simulink library "MOT_lib"  (R2016b)
settings: Solver=ode45  StartTime=0.0  StopTime=10.0  RelTol=1e-3  EnableMultiTasking=on
values from neighbouring files (symbols this model uses):
  MOT = MOTmod    [setup_mot.m]    (also in setup_motor.m)
undefined symbols (not defined in the file or in its folder): DiscIntNeverNeededParam
libraries: aerolibutil x1, aerolibtransform2 x1
settings Model: Creator=Andrew  LastModifiedBy=Andrew
settings DataIOCC: LimitDataPoints=on  SaveFormat=Array
settings OptimizationCC: LifeSpan=inf
settings DebuggingCC: SFUnexpectedBacktrackingDiag=warning  SFNoUnconditionalDefaultTransitionDiag=warning  SFExecutionAtInitializationDiag=none
settings HardwareCC: ProdBitPerPointer=32  ProdBitPerSizeT=32  ProdBitPerPtrDiffT=32  ProdLargestAtomicFloat=None  ProdIntDivRoundTo=Undefined  ProdEndianess=Unspecified  ProdWordSize=32  ProdHWDeviceType=32-bit Generic
settings ModelReferenceCC: PropagateSignalLabelsOutOfModel=off
settings GRTTargetCC: TargetLangStandard=C89/C90 (ANSI)  GeneratePreprocessorConditionals=Disable all
settings ConfigComp: CovMetricSettings=dw  CovHtmlReporting=on  CovSaveCumulativeToWorkspaceVar=on  CovSaveSingleToWorkspaceVar=on  CovExternalEMLEnable=off

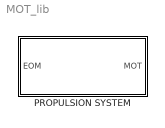
== system MOT_lib ==
  PROPULSION SYSTEM : Subsystem

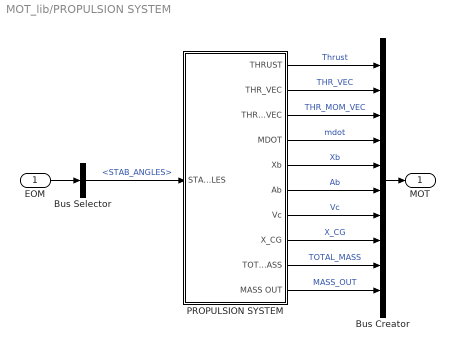
== system MOT_lib/PROPULSION SYSTEM ==
  EOM : Inport
  Bus Creator : BusCreator  Inputs=10
  Bus Selector : BusSelector  OutputSignals=STAB_ANGLES
  PROPULSION SYSTEM : Subsystem
  MOT : Outport
  wires:
  PROPULSION SYSTEM/1(THRUST) -> Bus Creator/1  "Thrust"
  PROPULSION SYSTEM/4(MDOT) -> Bus Creator/4  "mdot"
  Bus Creator/1 -> MOT/1
  PROPULSION SYSTEM/6(Ab) -> Bus Creator/6  "Ab"
  PROPULSION SYSTEM/10(MASS OUT) -> Bus Creator/10  "MASS_OUT"
  PROPULSION SYSTEM/5(Xb) -> Bus Creator/5  "Xb"
  PROPULSION SYSTEM/7(Vc) -> Bus Creator/7  "Vc"
  PROPULSION SYSTEM/8(X_CG) -> Bus Creator/8  "X_CG"
  PROPULSION SYSTEM/9(TOTAL_MASS) -> Bus Creator/9  "TOTAL_MASS"
  PROPULSION SYSTEM/3(THR_MOM_VEC) -> Bus Creator/3  "THR_MOM_VEC"
  PROPULSION SYSTEM/2(THR_VEC) -> Bus Creator/2  "THR_VEC"
  EOM/1 -> Bus Selector/1
  Bus Selector/1 -> PROPULSION SYSTEM/1(STAB_ANGLES)  "<STAB_ANGLES>"

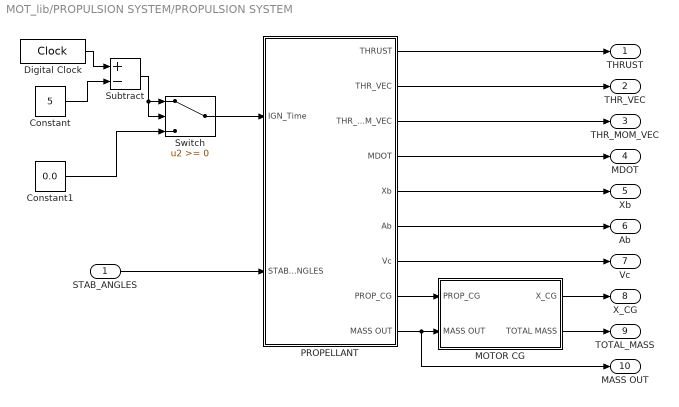
== system MOT_lib/PROPULSION SYSTEM/PROPULSION SYSTEM ==
  STAB_ANGLES : Inport
  Constant : Constant  Value=5
  Constant1 : Constant  Value=0.0
  Digital Clock : DigitalClock  SampleTime=0.0025
  MOTOR CG : Subsystem
  PROPELLANT : Subsystem
  Subtract : Sum  Inputs=+-
  Switch : Switch
  THRUST : Outport
  THR_VEC : Outport  Port=2
  THR_MOM_VEC : Outport  Port=3
  MDOT : Outport  Port=4
  Xb : Outport  Port=5
  Ab : Outport  Port=6
  Vc : Outport  Port=7
  X_CG : Outport  Port=8
  TOTAL_MASS : Outport  Port=9
  MASS OUT : Outport  Port=10
  wires:
  PROPELLANT/1(THRUST) -> THRUST/1
  PROPELLANT/4(MDOT) -> MDOT/1
  PROPELLANT/9(MASS OUT) -> MOTOR CG/2(MASS OUT), MASS OUT/1
  PROPELLANT/5(Xb) -> Xb/1
  PROPELLANT/6(Ab) -> Ab/1
  PROPELLANT/7(Vc) -> Vc/1
  PROPELLANT/8("PROP_CG ") -> MOTOR CG/1(PROP_CG)
  MOTOR CG/1(X_CG) -> X_CG/1
  MOTOR CG/2(TOTAL MASS) -> TOTAL_MASS/1
  PROPELLANT/2(THR_VEC) -> THR_VEC/1
  PROPELLANT/3(THR_MOM_VEC) -> THR_MOM_VEC/1
  STAB_ANGLES/1 -> PROPELLANT/2(STAB_ANGLES)
  Switch/1 -> PROPELLANT/1(IGN_Time)
  Digital Clock/1 -> Subtract/1
  Constant/1 -> Subtract/2
  Constant1/1 -> Switch/3
  Subtract/1 -> Switch/2, Switch/1

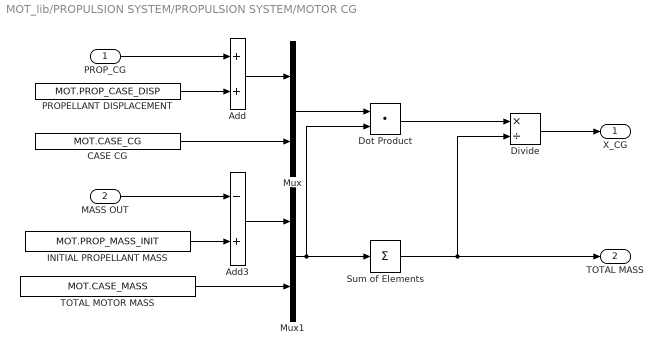
== system MOT_lib/PROPULSION SYSTEM/PROPULSION SYSTEM/MOTOR CG ==
  PROP_CG : Inport
  MASS OUT : Inport  Port=2
  Add : Sum
  Add3 : Sum  Inputs=-+
  CASE CG : Constant  Value=MOT.CASE_CG
  Divide : Product  Inputs=*/
  Dot Product : DotProduct  InputSameDT=on  OutDataTypeStr=Inherit: Inherit via internal rule
  INITIAL PROPELLANT MASS : Constant  Value=MOT.PROP_MASS_INIT
  Mux : Mux  Inputs=2
  Mux1 : Mux  Inputs=2
  PROPELLANT DISPLACEMENT : Constant  Value=MOT.PROP_CASE_DISP
  Sum of Elements : Sum  Inputs=+
  TOTAL MOTOR MASS : Constant  Value=MOT.CASE_MASS
  X_CG : Outport
  TOTAL MASS : Outport  Port=2
  wires:
  PROP_CG/1 -> Add/1
  PROPELLANT DISPLACEMENT/1 -> Add/2
  Add/1 -> Mux/1
  CASE CG/1 -> Mux/2
  Mux/1 -> Dot Product/1
  Mux1/1 -> Dot Product/2, Sum of Elements/1
  TOTAL MOTOR MASS/1 -> Mux1/2
  Add3/1 -> Mux1/1
  MASS OUT/1 -> Add3/1
  INITIAL PROPELLANT MASS/1 -> Add3/2
  Sum of Elements/1 -> Divide/2, TOTAL MASS/1
  Divide/1 -> X_CG/1
  Dot Product/1 -> Divide/1

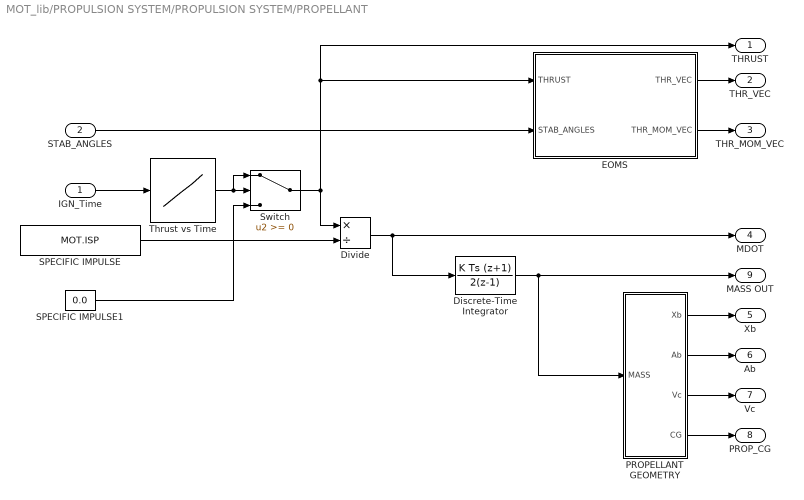
== system MOT_lib/PROPULSION SYSTEM/PROPULSION SYSTEM/PROPELLANT ==
  IGN_Time : Inport
  STAB_ANGLES : Inport  Port=2
  Discrete-Time Integrator : DiscreteIntegrator  IntegratorMethod=Integration: Trapezoidal  InitialConditionSetting=State (most efficient)  SampleTime=-1  ICPrevOutput=DiscIntNeverNeededParam  ICPrevScaledInput=DiscIntNeverNeededParam
  Divide : Product  Inputs=*/
  EOMS : Subsystem
  PROPELLANT GEOMETRY : Subsystem
  SPECIFIC IMPULSE : Constant  Value=MOT.ISP
  SPECIFIC IMPULSE1 : Constant  Value=0.0
  Switch : Switch
  Thrust vs Time : Lookup_n-D  NumberOfTableDimensions=1  BreakpointsForDimension1=MOT.THRUST_TABLE_X  Table=MOT.THRUST_TABLE_Y  InternalRulePriority=Speed  RndMeth=Simplest  InputSameDT=on
  THRUST : Outport
  THR_VEC : Outport  Port=2
  THR_MOM_VEC : Outport  Port=3
  MDOT : Outport  Port=4
  Xb : Outport  Port=5
  Ab : Outport  Port=6
  Vc : Outport  Port=7
  "PROP_CG " : Outport  Port=8
  MASS OUT : Outport  Port=9
  wires:
  PROPELLANT GEOMETRY/2(Ab) -> Ab/1
  Discrete-Time Integrator/1 -> PROPELLANT GEOMETRY/1(MASS), MASS OUT/1
  PROPELLANT GEOMETRY/3(Vc) -> Vc/1
  PROPELLANT GEOMETRY/4(CG) -> "PROP_CG "/1
  PROPELLANT GEOMETRY/1(Xb) -> Xb/1
  IGN_Time/1 -> Thrust vs Time/1
  SPECIFIC IMPULSE/1 -> Divide/2
  Divide/1 -> MDOT/1, Discrete-Time Integrator/1
  EOMS/1(THR_VEC) -> THR_VEC/1
  EOMS/2(THR_MOM_VEC) -> THR_MOM_VEC/1
  STAB_ANGLES/1 -> EOMS/2(STAB_ANGLES)
  Thrust vs Time/1 -> Switch/2, Switch/1
  Switch/1 -> THRUST/1, EOMS/1(THRUST), Divide/1
  SPECIFIC IMPULSE1/1 -> Switch/3

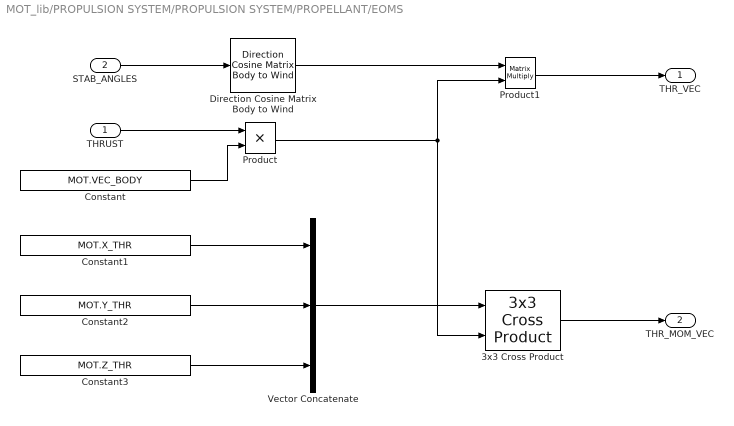
== system MOT_lib/PROPULSION SYSTEM/PROPULSION SYSTEM/PROPELLANT/EOMS ==
  THRUST : Inport
  STAB_ANGLES : Inport  Port=2
  3x3 Cross Product : aerolibutil/3x3 Cross Product
  Constant : Constant  Value=MOT.VEC_BODY
  Constant1 : Constant  Value=MOT.X_THR
  Constant2 : Constant  Value=MOT.Y_THR
  Constant3 : Constant  Value=MOT.Z_THR
  Direction Cosine Matrix Body to Wind : aerolibtransform2/Direction Cosine Matrix Body to Wind
  Product : Product
  Product1 : Product  Multiplication=Matrix(*)
  Vector Concatenate : Concatenate  NumInputs=3
  THR_VEC : Outport
  THR_MOM_VEC : Outport  Port=2
  wires:
  THRUST/1 -> Product/1
  Constant/1 -> Product/2
  Product/1 -> Product1/2, 3x3 Cross Product/2
  Constant1/1 -> Vector Concatenate/1
  Constant2/1 -> Vector Concatenate/2
  Constant3/1 -> Vector Concatenate/3
  Vector Concatenate/1 -> 3x3 Cross Product/1
  3x3 Cross Product/1 -> THR_MOM_VEC/1
  Direction Cosine Matrix Body to Wind/1 -> Product1/1
  Product1/1 -> THR_VEC/1
  STAB_ANGLES/1 -> Direction Cosine Matrix Body to Wind/1

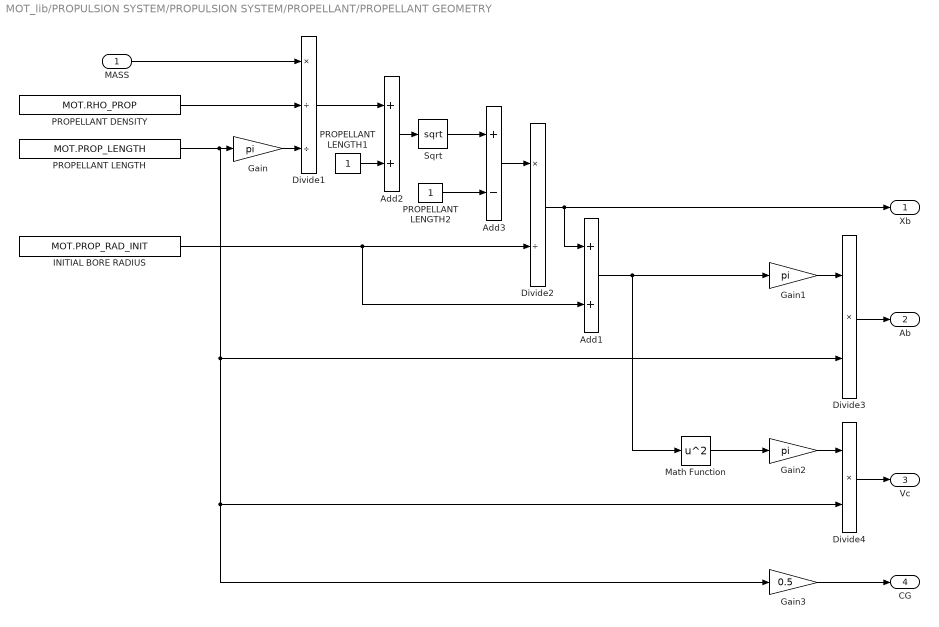
== system MOT_lib/PROPULSION SYSTEM/PROPULSION SYSTEM/PROPELLANT/PROPELLANT GEOMETRY ==
  MASS : Inport
  Add1 : Sum
  Add2 : Sum
  Add3 : Sum  Inputs=+-
  Divide1 : Product  Inputs=*//
  Divide2 : Product  Inputs=*/
  Divide3 : Product  Inputs=**
  Divide4 : Product  Inputs=**
  Gain : Gain  Gain=pi
  Gain1 : Gain  Gain=pi
  Gain2 : Gain  Gain=pi
  Gain3 : Gain  Gain=0.5
  INITIAL BORE RADIUS : Constant  Value=MOT.PROP_RAD_INIT
  Math Function : Math  Operator=square  SaturateOnIntegerOverflow=on
  PROPELLANT DENSITY : Constant  Value=MOT.RHO_PROP
  PROPELLANT LENGTH : Constant  Value=MOT.PROP_LENGTH
  PROPELLANT LENGTH1 : Constant
  PROPELLANT LENGTH2 : Constant
  Sqrt : Sqrt  SaturateOnIntegerOverflow=on
  Xb : Outport
  Ab : Outport  Port=2
  Vc : Outport  Port=3
  CG : Outport  Port=4
  wires:
  PROPELLANT DENSITY/1 -> Divide1/2
  Gain/1 -> Divide1/3
  Divide1/1 -> Add2/1
  Add2/1 -> Sqrt/1
  Sqrt/1 -> Add3/1
  PROPELLANT LENGTH2/1 -> Add3/2
  PROPELLANT LENGTH1/1 -> Add2/2
  PROPELLANT LENGTH/1 -> Divide3/2, Gain3/1, Divide4/2, Gain/1
  MASS/1 -> Divide1/1
  Add3/1 -> Divide2/1
  Divide2/1 -> Xb/1, Add1/1
  INITIAL BORE RADIUS/1 -> Add1/2, Divide2/2
  Add1/1 -> Gain1/1, Math Function/1
  Gain1/1 -> Divide3/1
  Divide3/1 -> Ab/1
  Divide4/1 -> Vc/1
  Gain2/1 -> Divide4/1
  Math Function/1 -> Gain2/1
  Gain3/1 -> CG/1
